simulink model "mppt_zero_handled"  (R2022a)
settings: Solver=VariableStepAuto  StartTime=0.0  StopTime=1.5  RelTol=1e-3
undefined symbols (not defined in the file or in its folder): DiscIntNeverNeededParam
libraries: simulink x5, spsSeriesRLCBranchLib x4, spsDiodeLib x2, fuzblock x2, spsIGBTDiodeLib x1, spsCurrentMeasurementLib x1, spsPVArrayLib x1, spsPWMGeneratorDCDCLib x1, spsVoltageMeasurementLib x1, spspowerguiLib x1
settings Model: Creator=IshaanKarnik  LastModifiedBy=IshaanKarnik
settings DebuggingCC: UnconnectedInputMsg=warning  UnconnectedOutputMsg=warning  UnconnectedLineMsg=warning
settings RTWCC: DLArmComputeVersion=19.05

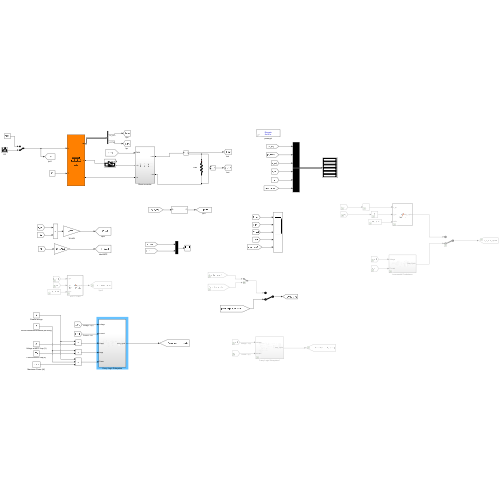
[thumbnail: Simulink's stored preview of the top-level diagram]
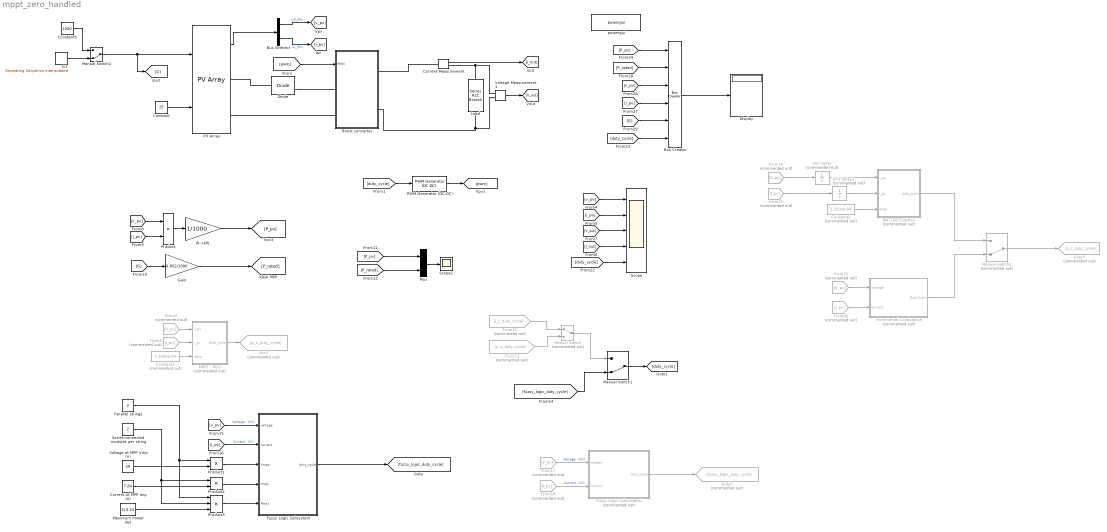
== system mppt_zero_handled ==
  Boost converter : Subsystem
  Bus Creator : BusCreator  Inputs=6
  Bus Selector : BusSelector  OutputSignals=V_PV,I_PV
  Constant : Constant  Value=25
  Constant1 : Constant  Commented=on  Value=1.2500e-04
  Constant2 : Constant  Commented=on  Value=1.2500e-04
  Constant3 : Constant  Value=1000
  Current Measurement : spsCurrentMeasurementLib/Current Measurement  PhasorSimulation=off  OutputType=Complex  PSBequivalent=0
  Current at MPP Imp (A) : Constant  Value=7.84
  Diode : spsDiodeLib/Diode  Ron=0.001  Lon=0  Vf=0.8  IC=0  UseSnubber=0  Rs=500  Cs=250e-9  Measurements=on
  Display : Display
  From13 : From  Commented=on  GotoTag=p_o_duty_cycle
  From{2,17,19,25} (4 alike) : From  Commented=on  GotoTag=V_pv
  From{3,18,20,30} (4 alike) : From  Commented=on  GotoTag=I_pv
  From21 : From  Commented=on  GotoTag=i_c_duty_cycle
  Fuzzy Logic Subsystem : Subsystem
  Fuzzy Logic Subsystem1 : Subsystem  Commented=on
  G2 : simulink/Sources/Repeating Sequence Interpolated  OutValues=[0 0 300 300 500 500 1000 1000 500 500 0 0].'  TimeValues=[0 0.25 0.2501 0.5 0.501 0.75 0.7501 1 1.01 1.25 1.2501 1.5].'  LookUpMeth=Interpolation-Use End Values  tsamp=0.01  OutMin=[]  OutMax=[]  OutDataTypeStr=double  OutputDataTypeScalingMode=double  OutDataType=fixdt(0,8)  OutScaling=2^-10
  Gain : Gain  Gain=0.852/1000
  Goto2 : Goto  Commented=on  GotoTag=fuzzy_logic_duty_cycle
  Goto4 : Goto  Commented=on  GotoTag=i_c_duty_cycle
  Incremental Condutance : Subsystem  Commented=on
  Load : spsSeriesRLCBranchLib/Series RLC Branch  LConnTagsString=__new0  RConnTagsString=__new0  BranchType=R  Resistance=20  Inductance=1e-3  SetiL0=off  InitialCurrent=0  Capacitance=100e-6  Setx0=off  InitialVoltage=0  Measurements=None
  MATLAB Function : MATLAB Function  Commented=on  TreatAsAtomicUnit=on
  MPPT - P&O : MATLAB Function  Commented=on  TreatAsAtomicUnit=on
  Manual Switch : ManualSwitch  Commented=on
  Manual Switch1 : ManualSwitch  CurrentSetting=0
  Manual Switch2 : ManualSwitch  CurrentSetting=0
  Manual Switch3 : ManualSwitch  Commented=on  CurrentSetting=0
  Maximum Power (W) : Constant  Value=213.15
  Mux : Mux  Inputs=2
  PV Array : spsPVArrayLib/PV Array  Npar=2  Nser=2  PlotType=array @ 25 deg.C & specified irradiances  S_vec="[ 1000  500  100 ]"  Temp_C_vec="[ 45 25  ]"  ModuleName=User-defined  PlotWhenSelected=off  Pm=213.15  Ncell=60  Voc=36.3  Isc=7.84  Vm=29  Im=7.35  beta_Voc_pc=-0.36099  alpha_Isc_pc=0.102  beta_Voc=-0.13104  alpha_Isc=0.0079968  IL=7.8654  I0=2.9273e-10  nI=0.98119  Rsh=313.0553  Rs=0.39381  RobustModel=off  RobustCellTemperature=313.3991  BAL=off  Tc=1e-6  Tfilter=5e-5
  PWM Generator (DC-DC) : spsPWMGeneratorDCDCLib/PWM Generator (DC-DC)  Fsw=5000  Ts=5e-6
  Parallel strings : Constant  Value=2
  Product : Product
  Product1 : Product
  Product2 : Product
  Product3 : Product  Inputs=3
  Scope : Scope  NumInputPorts=5
  Scope1 : Scope
  Series-connected modules per string : Constant  Value=2
  Unit Delay : UnitDelay  Commented=on  SampleTime=100e-6  HasFrameUpgradeWarning=on
  Unit Delay1 : UnitDelay  Commented=on  SampleTime=100e-6  HasFrameUpgradeWarning=on
  Voltage Measurement1 : spsVoltageMeasurementLib/Voltage Measurement  PhasorSimulation=off  OutputType=Complex  PSBequivalent=0
  Voltage at MPP Vmp (V) : Constant  Value=29
  Vpv2 : Goto  Commented=on  GotoTag=p_o_duty_cycle
  W->kW : Gain  Gain=1/1000
  powergui : spspowerguiLib/powergui  Priority=1  SimulationMode=Discrete  SampleTime=5e-6  frequency=60  Iterations=50  frequencyindice=0  Pbase=100e6  ErrMax=1e-4  UnitsV=kV  UnitsW=MW  buscounter=0  FunctionMessages=off  echomessages=off  EnableUseOfTLC=off  CurrentSourceSwitches=off  DisableSnubberDevices=off  DisableRonSwitches=off  DisableVfSwitches=off  DisplayEquations=off  AutomaticDiscreteSolvers=off  SolverType=Tustin/Backward Euler (TBE)  Interpol=off  ExternalGateDelay=off  methode=off  Ts=100  x0status=blocks  SPID=on  SwTol=0  HookPort=off  NonlinearTolerance=1e-4  nMaxIteration=100  ContinueOnMaxIteration=off  RestoreLinks=warning  ResistiveCurrentMeasurement=off  Frange=[0:2:500]  Ylog=off  Xlog=on  ShowGrid=off  save=off  variable=ZData  structure=0  ZoomFFT=off  StartTime=0.0  cycles=1  DisplayStyle=1  fundamental=60  FreqAxis=off  MaxFrequency=1000  frequencyindicesteady=1  RmsSteady=1  display=off
  wires:
  [I_out] -> Scope/4
  Unit Delay/1 -> MATLAB Function/1(v_pv)
  From25/1 -> Incremental Condutance/1(Voltage)
  [v_pv] -> Scope/1
  Manual Switch1/1 -> [duty_cycle]
  [duty_cycle] -> Scope/5
  [fuzzy_logic_duty_cycle] -> Manual Switch1/2
  Constant3/1 -> Manual Switch2/1
  From19/1 -> Unit Delay/1
  Bus Creator/1 -> Display/1
  Bus Selector/1 -> [v_pv]  "<V_PV>"
  Manual Switch2/1 -> [G], PV Array/1
  [v_pv] -> Product/1
  [G] -> Bus Creator/5
  Gain/1 -> [P_rated]
  [P_pv] -> Mux/1
  MPPT - P&O/1(duty_cycle) -> Vpv2/1
  [G] -> Gain/1
  [i_pv] -> Scope/2
  [P_rated] -> Bus Creator/2
  [duty_cycle] -> PWM Generator (DC-DC)/1
  W->kW/1 -> [P_pv]
  Constant/1 -> PV Array/2
  Bus Selector/2 -> [i_pv]  "<I_PV>"
  [i_pv] -> Product/2
  Product/1 -> W->kW/1
  Constant1/1 -> MPPT - P&O/3(delta)
  From13/1 -> Manual Switch/2
  Mux/1 -> Scope1/1
  [v_pv] -> Fuzzy Logic Subsystem/1(voltage)  "Voltage - V(n)"
  From3/1 -> MPPT - P&O/2(i_pv)
  From17/1 -> Fuzzy Logic Subsystem1/1(voltage)  "Voltage - V(n)"
  G2/1 -> Manual Switch2/2
  From21/1 -> Manual Switch/1
  Constant2/1 -> MATLAB Function/3(delta)
  From30/1 -> Incremental Condutance/2(Current)
  From2/1 -> MPPT - P&O/1(v_pv)
  Fuzzy Logic Subsystem1/1(duty_cycle) -> Goto2/1
  [pwm] -> Boost converter/1(PWM)
  Voltage Measurement1/1 -> [V_out]
  Unit Delay1/1 -> MATLAB Function/2(i_pv)
  MATLAB Function/1(duty_cycle) -> Manual Switch3/1
  [V_out] -> Scope/3
  [i_pv] -> Bus Creator/4
  [v_pv] -> Bus Creator/3
  Current Measurement/1 -> [I_out]
  From18/1 -> Fuzzy Logic Subsystem1/2(current)  "Current - I(n)"
  [P_rated] -> Mux/2
  PV Array/1 -> Bus Selector/1
  From20/1 -> Unit Delay1/1
  Manual Switch3/1 -> Goto4/1
  PWM Generator (DC-DC)/1 -> [pwm]
  [duty_cycle] -> Bus Creator/6
  [i_pv] -> Fuzzy Logic Subsystem/2(current)  "Current - I(n)"
  Incremental Condutance/1(Duty Cycle) -> Manual Switch3/2
  Manual Switch/1 -> Manual Switch1/1
  [P_pv] -> Bus Creator/1
  Fuzzy Logic Subsystem/1(duty_cycle) -> [fuzzy_logic_duty_cycle]
  Product1/1 -> Fuzzy Logic Subsystem/3(Vmpp)
  Voltage at MPP Vmp (V)/1 -> Product1/2
  Product2/1 -> Fuzzy Logic Subsystem/4(Impp)
  Current at MPP Imp (A)/1 -> Product2/2
  Product3/1 -> Fuzzy Logic Subsystem/5(Pmax)
  Series-connected modules per string/1 -> Product3/2, Product2/1
  Parallel strings/1 -> Product3/1, Product1/1
  Maximum Power (W)/1 -> Product3/3
  connections:
  Boost converter/RConn2 -- Voltage Measurement1/LConn2 -- Load/RConn1
  Current Measurement/RConn1 -- Voltage Measurement1/LConn1 -- Load/LConn1
  PV Array/RConn2 -- Boost converter/LConn2
  Current Measurement/LConn1 -- Boost converter/RConn1
  Diode/RConn1 -- Boost converter/LConn1
  Diode/LConn1 -- PV Array/RConn1

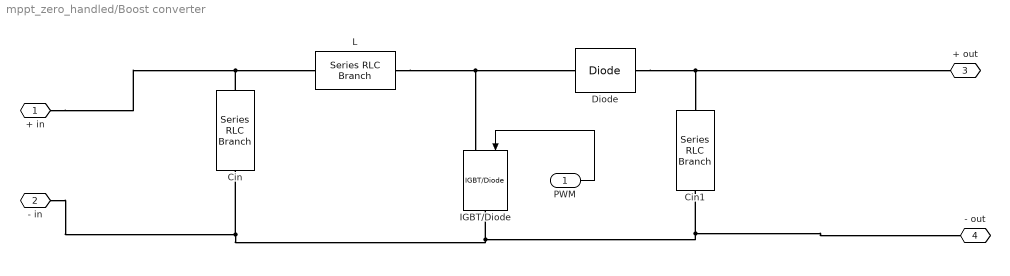
== system mppt_zero_handled/Boost converter ==
  PWM : Inport
  Cin : spsSeriesRLCBranchLib/Series RLC Branch  LConnTagsString=__new0  RConnTagsString=__new0  BranchType=RC  Resistance=1e-3  Inductance=1e-3  SetiL0=off  InitialCurrent=0  Capacitance=50e-6  Setx0=off  InitialVoltage=0  Measurements=None
  Cin1 : spsSeriesRLCBranchLib/Series RLC Branch  LConnTagsString=__new0  RConnTagsString=__new0  BranchType=RC  Resistance=1e-4  Inductance=1e-3  SetiL0=off  InitialCurrent=0  Capacitance=10e-6  Setx0=off  InitialVoltage=0  Measurements=None
  Diode : spsDiodeLib/Diode  Ron=0.001  Lon=0  Vf=0.8  IC=0  UseSnubber=0  Rs=500  Cs=250e-9  Measurements=off
  IGBT/Diode : spsIGBTDiodeLib/IGBT//Diode  Ron=1e-3  Rs=1e5  Cs=inf  Measurements=off
  L : spsSeriesRLCBranchLib/Series RLC Branch  LConnTagsString=__new0  RConnTagsString=__new0  BranchType=RL  Resistance=0.1  Inductance=2e-3  SetiL0=off  InitialCurrent=0  Capacitance=100e-6  Setx0=off  InitialVoltage=0  Measurements=None
  + in : PMIOPort  Side=Left
  - in : PMIOPort  Port=2  Side=Left
  + out : PMIOPort  Port=3  Side=Right
  - out : PMIOPort  Port=4  Side=Right
  wires:
  PWM/1 -> IGBT/Diode/1
  connections:
  Cin/LConn1 -- + in/RConn1 -- L/RConn1
  - in/RConn1 -- Cin/RConn1 -- - out/RConn1 -- Cin1/RConn1 -- IGBT/Diode/RConn1
  L/LConn1 -- Diode/LConn1 -- IGBT/Diode/LConn1
  Diode/RConn1 -- + out/RConn1 -- Cin1/LConn1

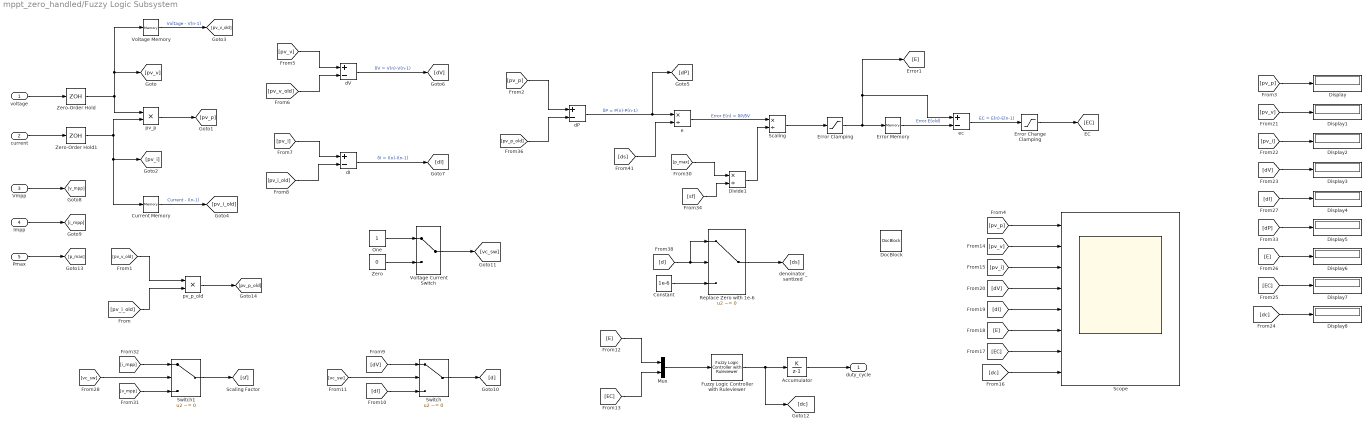
== system mppt_zero_handled/Fuzzy Logic Subsystem ==
  voltage : Inport
  current : Inport  Port=2
  Vmpp : Inport  Port=3
  Impp : Inport  Port=4
  Pmax : Inport  Port=5
  Accumulator : DiscreteIntegrator  IntegratorMethod=Accumulation: Forward Euler  gainval=0.1  InitialCondition=0.3  SampleTime=-1  LimitOutput=on  UpperSaturationLimit=1  LowerSaturationLimit=0  ICPrevOutput=DiscIntNeverNeededParam  ICPrevScaledInput=DiscIntNeverNeededParam
  Constant : Constant  Value=1e-6
  Current Memory : Memory
  Display{,1..8} (9 alike) : Display
  Divide1 : Product  Inputs=*/
  DocBlock : simulink/Model-Wide Utilities/DocBlock  DocumentType=Text
      content=|
      | Error E(n) = δP/δV or
      | Error E(n) = δP/δI
      | Depending on the manual switch setting
  Error Change Clamping : Saturate  UpperLimit=2  LowerLimit=-2
  Error Clamping : Saturate  UpperLimit=1  LowerLimit=-1
  Error Memory : Memory
  Fuzzy Logic Controller with Ruleviewer : fuzblock/Fuzzy Logic  Controller  with Ruleviewer  fismatrix=fuzzy_mppt  Ts=0.1
  Mux : Mux  Inputs=2
  One : Constant  OutDataTypeStr=Inherit: Inherit via back propagation
  Replace Zero with 1e-6 : Switch  Criteria=u2 ~= 0  SaturateOnIntegerOverflow=off  InputSameDT=off
  Scaling : Product  Inputs=*/
  Scope : Scope  NumInputPorts=8
  Switch : Switch  Criteria=u2 ~= 0  SaturateOnIntegerOverflow=off  InputSameDT=off
  Switch1 : Switch  Criteria=u2 ~= 0  SaturateOnIntegerOverflow=off  InputSameDT=off
  Voltage Current Switch : ManualSwitch
  Voltage Memory : Memory
  Zero : Constant  Value=0  OutDataTypeStr=Inherit: Inherit via back propagation
  Zero-Order Hold : ZeroOrderHold  SampleTime=-1
  Zero-Order Hold1 : ZeroOrderHold  SampleTime=-1
  dI : Sum  Inputs=+-
  dP : Sum  Inputs=+-
  dV : Sum  Inputs=+-
  e : Product  Inputs=*/
  ec : Sum  Inputs=+-
  pv_p : Product
  pv_p_old : Product
  duty_cycle : Outport
  wires:
  ec/1 -> Error Change Clamping/1  "EC = E(n)-E(n-1)"
  dP/1 -> [dP], e/1  "δP = P(n)-P(n-1)"
  [dI] -> Display4/1
  dV/1 -> [dV]  "δV = V(n)-V(n-1)"
  [EC] -> Display7/1
  Voltage Memory/1 -> [pv_v_old]  "Voltage - V(n-1)"
  [pv_v_old] -> dV/2
  [pv_i_old] -> dI/2
  [pv_v] -> dV/1
  [EC] -> Mux/2
  [pv_i] -> Display2/1
  dI/1 -> [dI]  "δI = I(n)-I(n-1)"
  Error Memory/1 -> ec/2  "Error E(old)"
  [pv_p] -> Scope/1
  [pv_p] -> Display/1
  [dV] -> Scope/4
  [pv_i] -> Scope/3
  [E] -> Display6/1
  [pv_v] -> Scope/2
  [dI] -> Scope/5
  [dc] -> Display8/1
  [E] -> Mux/1
  Current Memory/1 -> [pv_i_old]  "Current - I(n-1)"
  [dc] -> Scope/8
  [EC] -> Scope/7
  [E] -> Scope/6
  [pv_i] -> dI/1
  [dV] -> Display3/1
  [pv_v] -> Display1/1
  current/1 -> Zero-Order Hold1/1
  voltage/1 -> Zero-Order Hold/1
  Zero-Order Hold1/1 -> Current Memory/1, [pv_i], pv_p/2
  Zero-Order Hold/1 -> pv_p/1, Voltage Memory/1, [pv_v]
  [dP] -> Display5/1
  pv_p/1 -> [pv_p]
  [pv_v_old] -> pv_p_old/1
  [pv_i_old] -> pv_p_old/2
  pv_p_old/1 -> [pv_p_old]
  [pv_p_old] -> dP/2
  [pv_p] -> dP/1
  Error Change Clamping/1 -> [EC]
  Vmpp/1 -> [v_mpp]
  Impp/1 -> [i_mpp]
  Pmax/1 -> [p_max]
  e/1 -> Scaling/1  "Error E(n) = δP/δV"
  [sf] -> Divide1/2
  Mux/1 -> Fuzzy Logic Controller with Ruleviewer/1
  [p_max] -> Divide1/1
  Constant/1 -> Replace Zero with 1e-6/3
  [d] -> Replace Zero with 1e-6/2, Replace Zero with 1e-6/1
  Replace Zero with 1e-6/1 -> [ds]
  [ds] -> e/2
  Scaling/1 -> Error Clamping/1
  Error Clamping/1 -> ec/1, [E], Error Memory/1
  Accumulator/1 -> duty_cycle/1
  Fuzzy Logic Controller with Ruleviewer/1 -> [dc], Accumulator/1
  Switch/1 -> [d]
  [dV] -> Switch/1
  [dI] -> Switch/3
  Switch1/1 -> [sf]
  Zero/1 -> Voltage Current Switch/2
  One/1 -> Voltage Current Switch/1
  Voltage Current Switch/1 -> [vc_sw]
  [vc_sw] -> Switch1/2
  [vc_sw] -> Switch/2
  Divide1/1 -> Scaling/2
  [v_mpp] -> Switch1/3
  [i_mpp] -> Switch1/1

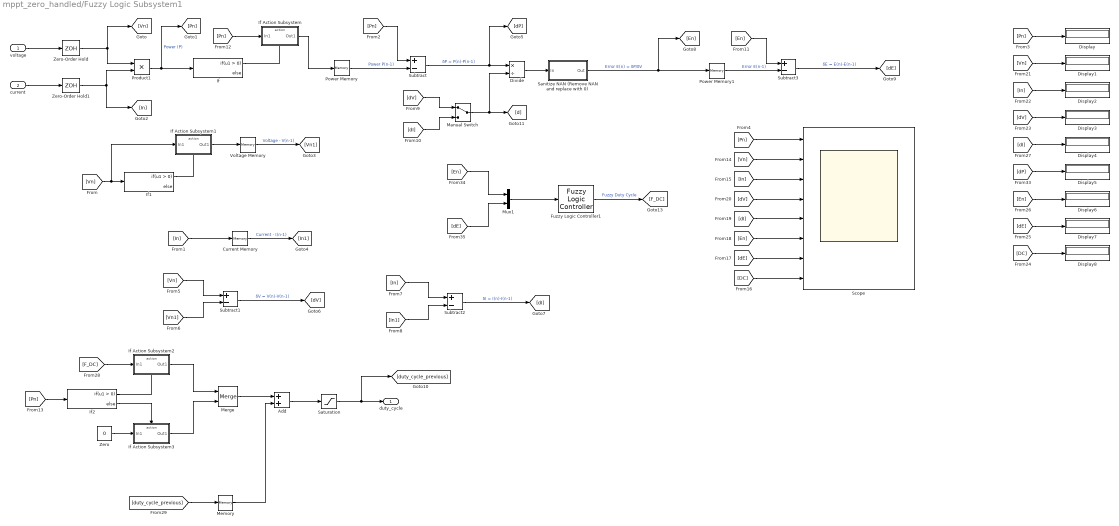
== system mppt_zero_handled/Fuzzy Logic Subsystem1 ==
  voltage : Inport
  current : Inport  Port=2
  Add : Sum
  Current Memory : Memory
  Display{,1..8} (9 alike) : Display
  Divide : Product  Inputs=*/
  Fuzzy Logic Controller1 : fuzblock/Fuzzy Logic  Controller  FIS=fuzzy_mppt  OutputSampleNumber=101  DataType=double  FuzzifiedInputs=off  RuleFiringStrengths=off  RuleOutputs=off  AggregatedOutputs=off  SimulateUsing=Interpreted execution  OutOfRangeInputValueMessage=warning  NoRuleFiredMessage=warning  EmptyOutputFuzzySetMessage=warning
  If : If
  If Action Subsystem : Subsystem  TreatAsAtomicUnit=on
  If Action Subsystem1 : Subsystem  TreatAsAtomicUnit=on
  If Action Subsystem2 : Subsystem  TreatAsAtomicUnit=on
  If Action Subsystem3 : Subsystem  TreatAsAtomicUnit=on
  If1 : If
  If2 : If
  Manual Switch : ManualSwitch
  Memory : Memory
  Merge : Merge
  Mux1 : Mux  Inputs=2
  Power Memory : Memory
  Power Memory1 : Memory
  Product1 : Product
  Sanitize NAN (Remove NAN and replace with 0) : Subsystem
  Saturation : Saturate  UpperLimit=0.85  LowerLimit=0
  Scope : Scope  NumInputPorts=8
  Subtract{,1..3} (4 alike) : Sum  Inputs=+-
  Voltage Memory : Memory
  Zero : Constant  Value=0  OutDataTypeStr=Inherit: Inherit via back propagation
  Zero-Order Hold : ZeroOrderHold  SampleTime=-1
  Zero-Order Hold1 : ZeroOrderHold  SampleTime=-1
  duty_cycle : Outport
  wires:
  Sanitize NAN (Remove NAN and replace with 0)/1(Out) -> [En], Power Memory1/1  "Error E(n) = δP/δV"
  Subtract3/1 -> [dE]  "δE = E(n)-E(n-1)"
  Subtract/1 -> [dP], Divide/1  "δP = P(n)-P(n-1)"
  [Pn] -> Subtract/1
  [dI] -> Display4/1
  Subtract1/1 -> [dV]  "δV = V(n)-V(n-1)"
  [dE] -> Display7/1
  Manual Switch/1 -> [d], Divide/2
  Voltage Memory/1 -> [Vn1]  "Voltage - V(n-1)"
  [Vn1] -> Subtract1/2
  [In1] -> Subtract2/2
  [Vn] -> Subtract1/1
  Power Memory/1 -> Subtract/2  "Power P(n-1)"
  [In] -> Display2/1
  Subtract2/1 -> [dI]  "δI = I(n)-I(n-1)"
  Power Memory1/1 -> Subtract3/2  "Error E(n-1)"
  [dV] -> Manual Switch/1
  [Pn] -> Scope/1
  [Pn] -> Display/1
  [dV] -> Scope/4
  [In] -> Scope/3
  [En] -> Display6/1
  [Vn] -> Scope/2
  [dI] -> Scope/5
  [En] -> Subtract3/1
  [DC] -> Display8/1
  Current Memory/1 -> [In1]  "Current - I(n-1)"
  [DC] -> Scope/8
  [dE] -> Scope/7
  [En] -> Scope/6
  [In] -> Subtract2/1
  [dV] -> Display3/1
  [dI] -> Manual Switch/2
  [Vn] -> Display1/1
  Memory/1 -> Add/2
  [duty_cycle_previous] -> Memory/1
  current/1 -> Zero-Order Hold1/1
  voltage/1 -> Zero-Order Hold/1
  Zero-Order Hold1/1 -> [In], Product1/2
  Zero-Order Hold/1 -> Product1/1, [Vn]
  [dP] -> Display5/1
  [En] -> Mux1/1
  Fuzzy Logic Controller1/1 -> [F_DC]  "Fuzzy Duty Cycle"
  Mux1/1 -> Fuzzy Logic Controller1/1
  [dE] -> Mux1/2
  Add/1 -> Saturation/1
  Saturation/1 -> [duty_cycle_previous], duty_cycle/1
  [In] -> Current Memory/1
  Divide/1 -> Sanitize NAN (Remove NAN and replace with 0)/1(In)
  Product1/1 -> If/1, [Pn]  "Power (P)"
  If/1 -> If Action Subsystem/Action
  If Action Subsystem/1(Out1) -> Power Memory/1
  [Pn] -> If Action Subsystem/1(In1)
  [Vn] -> If Action Subsystem1/1(In1), If1/1
  If Action Subsystem1/1(Out1) -> Voltage Memory/1
  If1/1 -> If Action Subsystem1/Action
  If2/1 -> If Action Subsystem2/Action
  [Pn] -> If2/1
  [F_DC] -> If Action Subsystem2/1(In1)
  Merge/1 -> Add/1
  If Action Subsystem2/1(Out1) -> Merge/1
  If2/2 -> If Action Subsystem3/Action
  If Action Subsystem3/1(Out1) -> Merge/2
  Zero/1 -> If Action Subsystem3/1(In1)

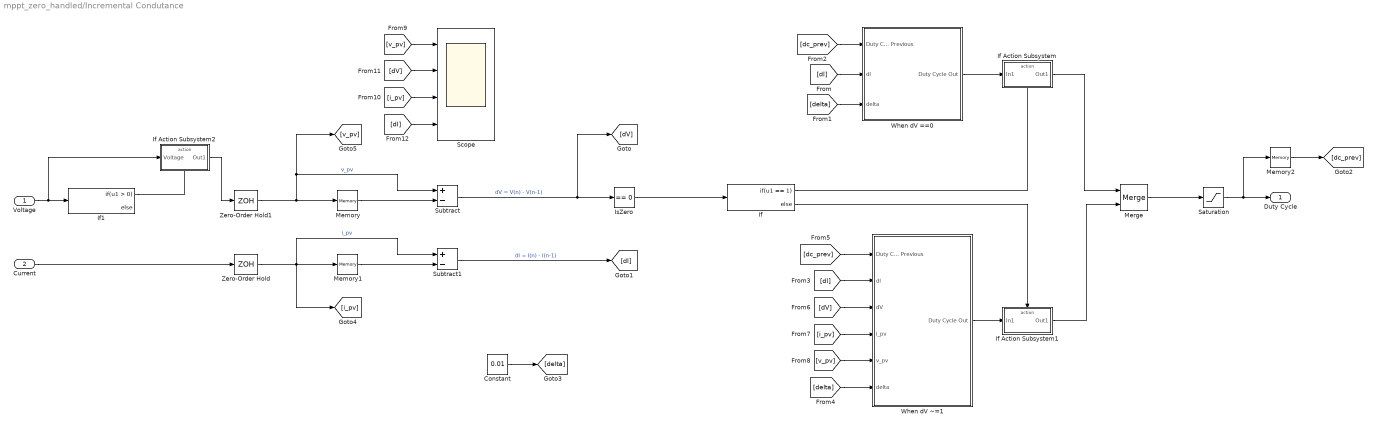
== system mppt_zero_handled/Incremental Condutance ==
  Voltage : Inport
  Current : Inport  Port=2
  Constant : Constant  Value=0.01
  If : If  IfExpression=u1 == 1
  If Action Subsystem : Subsystem  TreatAsAtomicUnit=on
  If Action Subsystem1 : Subsystem  TreatAsAtomicUnit=on
  If Action Subsystem2 : Subsystem  TreatAsAtomicUnit=on
  If1 : If
  IsZero : simulink/Logic and Bit Operations/Compare To Zero  relop===  OutDataTypeStr=boolean
  Memory : Memory
  Memory1 : Memory
  Memory2 : Memory
  Merge : Merge
  Saturation : Saturate  UpperLimit=0.85  LowerLimit=0
  Scope : Scope  NumInputPorts=4
  Subtract : Sum  Inputs=+-
  Subtract1 : Sum  Inputs=+-
  When dV ==0 : Subsystem
  When dV ~=1 : Subsystem
  Zero-Order Hold : ZeroOrderHold  SampleTime=-1
  Zero-Order Hold1 : ZeroOrderHold  SampleTime=-1
  Duty Cycle : Outport
  wires:
  Zero-Order Hold1/1 -> [v_pv], Subtract/1, Memory/1  "v_pv"
  Zero-Order Hold/1 -> [i_pv], Subtract1/1, Memory1/1  "i_pv"
  Memory/1 -> Subtract/2
  Memory1/1 -> Subtract1/2
  Subtract/1 -> [dV], IsZero/1  "dV = V(n) - V(n-1)"
  Subtract1/1 -> [dI]  "dI = I(n) - I(n-1)"
  IsZero/1 -> If/1
  If/2 -> If Action Subsystem1/Action
  If/1 -> If Action Subsystem/Action
  If Action Subsystem1/1(Out1) -> Merge/2
  Saturation/1 -> Memory2/1, Duty Cycle/1
  Memory2/1 -> [dc_prev]
  Constant/1 -> [delta]
  If Action Subsystem/1(Out1) -> Merge/1
  When dV ==0/1(Duty Cycle Out) -> If Action Subsystem/1(In1)
  [dI] -> When dV ==0/2(dI)
  [delta] -> When dV ==0/3(delta)
  [dc_prev] -> When dV ==0/1(Duty Cycle Previous)
  When dV ~=1/1(Duty Cycle Out) -> If Action Subsystem1/1(In1)
  Merge/1 -> Saturation/1
  [dc_prev] -> When dV ~=1/1(Duty Cycle Previous)
  [dI] -> When dV ~=1/2(dI)
  [dV] -> When dV ~=1/3(dV)
  [delta] -> When dV ~=1/6(delta)
  [i_pv] -> When dV ~=1/4(i_pv)
  [v_pv] -> When dV ~=1/5(v_pv)
  [v_pv] -> Scope/1
  [dV] -> Scope/2
  [i_pv] -> Scope/3
  [dI] -> Scope/4
  Voltage/1 -> If Action Subsystem2/1(Voltage), If1/1
  If1/1 -> If Action Subsystem2/Action
  If Action Subsystem2/1(Out1) -> Zero-Order Hold1/1
  Current/1 -> Zero-Order Hold/1

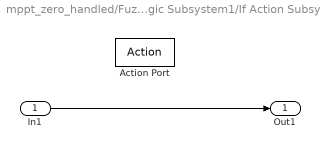
== system mppt_zero_handled/Fuzzy Logic Subsystem1/If Action Subsystem ==
  In1 : Inport
  Action Port : ActionPort
  Out1 : Outport
  wires:
  In1/1 -> Out1/1

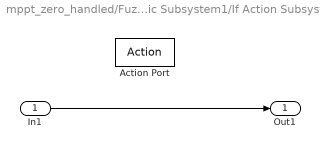
== system mppt_zero_handled/Fuzzy Logic Subsystem1/If Action Subsystem1 ==
  In1 : Inport
  Action Port : ActionPort
  Out1 : Outport
  wires:
  In1/1 -> Out1/1

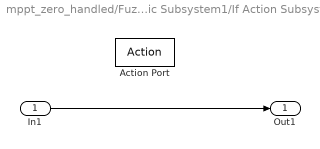
== system mppt_zero_handled/Fuzzy Logic Subsystem1/If Action Subsystem2 ==
  In1 : Inport
  Action Port : ActionPort
  Out1 : Outport
  wires:
  In1/1 -> Out1/1

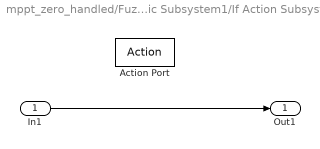
== system mppt_zero_handled/Fuzzy Logic Subsystem1/If Action Subsystem3 ==
  In1 : Inport
  Action Port : ActionPort
  Out1 : Outport
  wires:
  In1/1 -> Out1/1

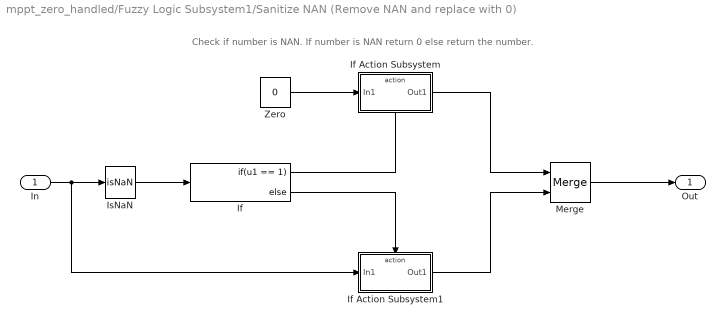
== system mppt_zero_handled/Fuzzy Logic Subsystem1/Sanitize NAN (Remove NAN and replace with 0) ==
  note: Check if number is NAN. If number is NAN return 0 else return the number.
  In : Inport
  If : If  IfExpression=u1 == 1
  If Action Subsystem : Subsystem  TreatAsAtomicUnit=on
  If Action Subsystem1 : Subsystem  TreatAsAtomicUnit=on
  IsNaN : RelationalOperator  Operator=isNaN  OutDataTypeStr=boolean  RndMeth=Simplest  InputSameDT=off
  Merge : Merge  InitialOutput=[0]
  Zero : Constant  Value=0  OutDataTypeStr=Inherit: Inherit via back propagation
  Out : Outport
  wires:
  If/1 -> If Action Subsystem/Action
  If Action Subsystem/1(Out1) -> Merge/1
  Zero/1 -> If Action Subsystem/1(In1)
  IsNaN/1 -> If/1
  In/1 -> If Action Subsystem1/1(In1), IsNaN/1
  Merge/1 -> Out/1
  If Action Subsystem1/1(Out1) -> Merge/2
  If/2 -> If Action Subsystem1/Action

== system mppt_zero_handled/Incremental Condutance/If Action Subsystem ==
  In1 : Inport
  Action Port : ActionPort
  Out1 : Outport
  wires:
  In1/1 -> Out1/1

== system mppt_zero_handled/Incremental Condutance/If Action Subsystem1 ==
  In1 : Inport
  Action Port : ActionPort
  Out1 : Outport
  wires:
  In1/1 -> Out1/1

== system mppt_zero_handled/Incremental Condutance/If Action Subsystem2 ==
  Voltage : Inport
  Action Port : ActionPort
  Out1 : Outport
  wires:
  Voltage/1 -> Out1/1

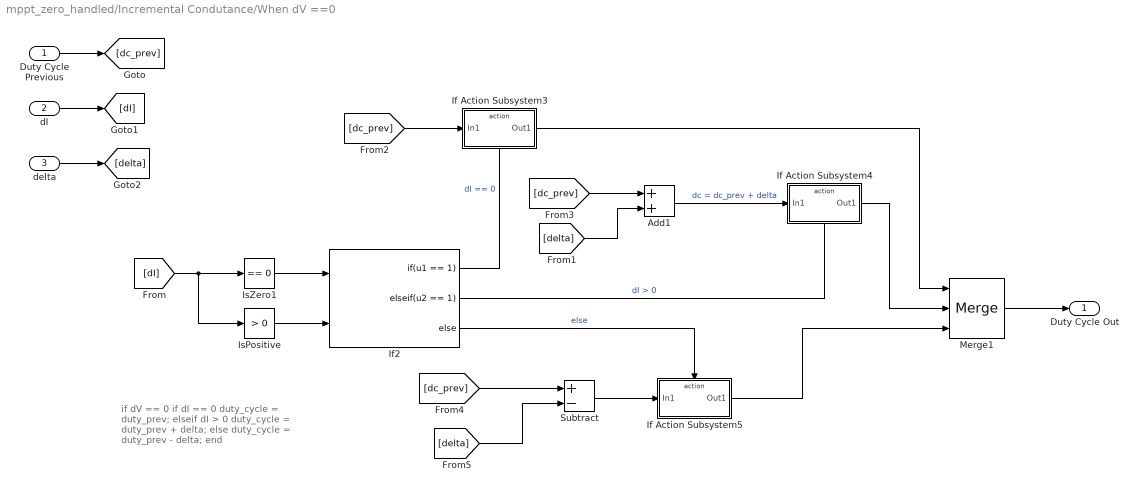
== system mppt_zero_handled/Incremental Condutance/When dV ==0 ==
  note: if dV == 0
      |     if dI == 0
      |         duty_cycle = duty_prev;
      |     elseif dI > 0
      |         duty_cycle = duty_prev + delta;
      |     else
      |         duty_cycle = duty_prev - delta;
      | end
  Duty Cycle Previous : Inport
  dI : Inport  Port=2
  delta : Inport  Port=3
  Add1 : Sum
  If Action Subsystem3 : Subsystem  TreatAsAtomicUnit=on
  If Action Subsystem4 : Subsystem  TreatAsAtomicUnit=on
  If Action Subsystem5 : Subsystem  TreatAsAtomicUnit=on
  If2 : If  NumInputs=2  IfExpression=u1 == 1  ElseIfExpressions=u2 == 1
  IsPositive : simulink/Logic and Bit Operations/Compare To Zero  relop=>  OutDataTypeStr=boolean
  IsZero1 : simulink/Logic and Bit Operations/Compare To Zero  relop===  OutDataTypeStr=boolean
  Merge1 : Merge  Inputs=3
  Subtract : Sum  Inputs=+-
  Duty Cycle Out : Outport
  wires:
  [dI] -> IsPositive/1, IsZero1/1
  IsZero1/1 -> If2/1
  Add1/1 -> If Action Subsystem4/1(In1)  "dc = dc_prev + delta"
  Subtract/1 -> If Action Subsystem5/1(In1)
  If2/3 -> If Action Subsystem5/Action  "else"
  [dc_prev] -> Add1/1
  If2/2 -> If Action Subsystem4/Action  "dI > 0"
  [dc_prev] -> Subtract/1
  If Action Subsystem3/1(Out1) -> Merge1/1
  [delta] -> Subtract/2
  IsPositive/1 -> If2/2
  Merge1/1 -> Duty Cycle Out/1
  If Action Subsystem5/1(Out1) -> Merge1/3
  If Action Subsystem4/1(Out1) -> Merge1/2
  [dc_prev] -> If Action Subsystem3/1(In1)
  If2/1 -> If Action Subsystem3/Action  "dI == 0"
  Duty Cycle Previous/1 -> [dc_prev]
  dI/1 -> [dI]
  delta/1 -> [delta]
  [delta] -> Add1/2

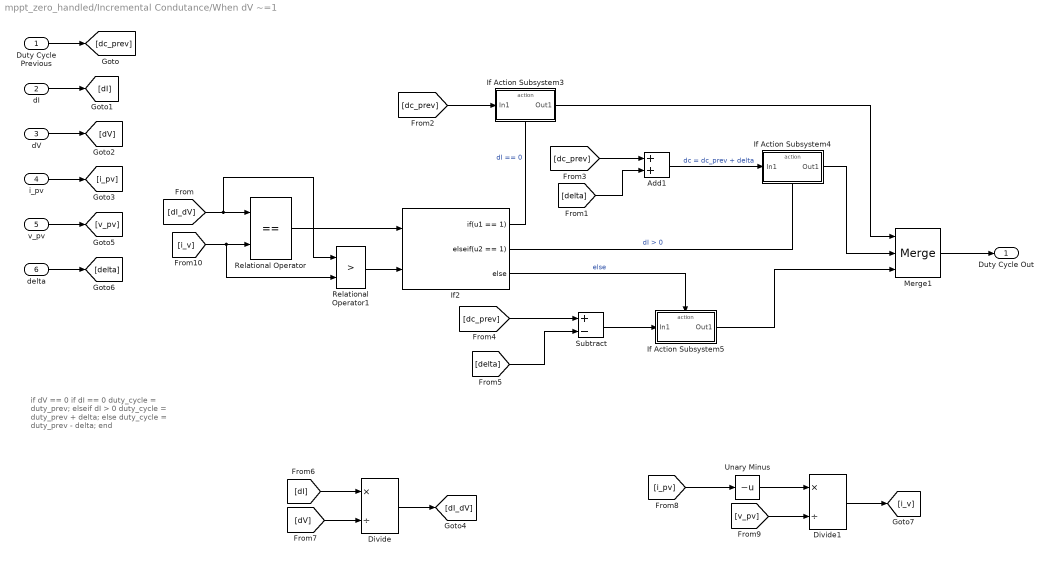
== system mppt_zero_handled/Incremental Condutance/When dV ~=1 ==
  note: if dV == 0
      |     if dI == 0
      |         duty_cycle = duty_prev;
      |     elseif dI > 0
      |         duty_cycle = duty_prev + delta;
      |     else
      |         duty_cycle = duty_prev - delta;
      | end
  Duty Cycle Previous : Inport
  dI : Inport  Port=2
  dV : Inport  Port=3
  i_pv : Inport  Port=4
  v_pv : Inport  Port=5
  delta : Inport  Port=6
  Add1 : Sum
  Divide : Product  Inputs=*/
  Divide1 : Product  Inputs=*/
  If Action Subsystem3 : Subsystem  TreatAsAtomicUnit=on
  If Action Subsystem4 : Subsystem  TreatAsAtomicUnit=on
  If Action Subsystem5 : Subsystem  TreatAsAtomicUnit=on
  If2 : If  NumInputs=2  IfExpression=u1 == 1  ElseIfExpressions=u2 == 1
  Merge1 : Merge  Inputs=3
  Relational Operator : RelationalOperator  Operator===  OutDataTypeStr=boolean  RndMeth=Simplest  InputSameDT=off
  Relational Operator1 : RelationalOperator  Operator=>  OutDataTypeStr=boolean  RndMeth=Simplest  InputSameDT=off
  Subtract : Sum  Inputs=+-
  Unary Minus : UnaryMinus
  Duty Cycle Out : Outport
  wires:
  [delta] -> Add1/2
  dV/1 -> [dV]
  dI/1 -> [dI]
  Duty Cycle Previous/1 -> [dc_prev]
  If2/1 -> If Action Subsystem3/Action  "dI == 0"
  [dc_prev] -> If Action Subsystem3/1(In1)
  If Action Subsystem4/1(Out1) -> Merge1/2
  If Action Subsystem5/1(Out1) -> Merge1/3
  Merge1/1 -> Duty Cycle Out/1
  [delta] -> Subtract/2
  If Action Subsystem3/1(Out1) -> Merge1/1
  [dc_prev] -> Subtract/1
  If2/2 -> If Action Subsystem4/Action  "dI > 0"
  [dc_prev] -> Add1/1
  If2/3 -> If Action Subsystem5/Action  "else"
  Subtract/1 -> If Action Subsystem5/1(In1)
  Add1/1 -> If Action Subsystem4/1(In1)  "dc = dc_prev + delta"
  i_pv/1 -> [i_pv]
  [dI] -> Divide/1
  [dV] -> Divide/2
  Divide/1 -> [dI_dV]
  v_pv/1 -> [v_pv]
  delta/1 -> [delta]
  [v_pv] -> Divide1/2
  [i_pv] -> Unary Minus/1
  Unary Minus/1 -> Divide1/1
  Divide1/1 -> [i_v]
  Relational Operator/1 -> If2/1
  [i_v] -> Relational Operator1/2, Relational Operator/2
  Relational Operator1/1 -> If2/2
  [dI_dV] -> Relational Operator1/1, Relational Operator/1

== system mppt_zero_handled/Fuzzy Logic Subsystem1/Sanitize NAN (Remove NAN and replace with 0)/If Action Subsystem ==
  In1 : Inport
  Action Port : ActionPort
  Out1 : Outport
  wires:
  In1/1 -> Out1/1

== system mppt_zero_handled/Fuzzy Logic Subsystem1/Sanitize NAN (Remove NAN and replace with 0)/If Action Subsystem1 ==
  In1 : Inport
  Action Port : ActionPort
  Out1 : Outport
  wires:
  In1/1 -> Out1/1

== system mppt_zero_handled/Incremental Condutance/When dV ==0/If Action Subsystem3 ==
  In1 : Inport
  Action Port : ActionPort
  Out1 : Outport
  wires:
  In1/1 -> Out1/1

== system mppt_zero_handled/Incremental Condutance/When dV ==0/If Action Subsystem4 ==
  In1 : Inport
  Action Port : ActionPort
  Out1 : Outport
  wires:
  In1/1 -> Out1/1

== system mppt_zero_handled/Incremental Condutance/When dV ==0/If Action Subsystem5 ==
  In1 : Inport
  Action Port : ActionPort
  Out1 : Outport
  wires:
  In1/1 -> Out1/1

== system mppt_zero_handled/Incremental Condutance/When dV ~=1/If Action Subsystem3 ==
  In1 : Inport
  Action Port : ActionPort
  Out1 : Outport
  wires:
  In1/1 -> Out1/1

== system mppt_zero_handled/Incremental Condutance/When dV ~=1/If Action Subsystem4 ==
  In1 : Inport
  Action Port : ActionPort
  Out1 : Outport
  wires:
  In1/1 -> Out1/1

== system mppt_zero_handled/Incremental Condutance/When dV ~=1/If Action Subsystem5 ==
  In1 : Inport
  Action Port : ActionPort
  Out1 : Outport
  wires:
  In1/1 -> Out1/1

== matlab function mppt_zero_handled/MATLAB Function ==
  data: v_pv input; duty_cycle output; i_pv input; delta input
function duty_cycle = mppt_i_c(v_pv, i_pv, delta)

duty_min=0;
duty_max=0.85;

persistent v_prev i_prev duty_prev;

if isempty(v_prev)
    v_prev = 0;
    i_prev = 0;
    duty_prev = 0.1;
end

dV = v_pv - v_prev;
dI = i_pv - i_prev;


%     if v_pv > 30
if dV == 0
    if dI == 0
        duty_cycle = duty_prev;
    elseif dI > 0
        duty_cycle = duty_prev + delta;
    else
        duty_cycle = duty_prev - delta;
    end
else
    if dI/dV == (-i_pv/v_pv)
        duty_cycle = duty_prev;
    elseif dI/dV > (-i_pv/v_pv)
        duty_cycle = duty_prev + delta;
    else
        duty_cycle = duty_prev - delta;
    end
end
%         duty_prev = duty_cycle;
%         v_prev = v_pv;
%         i_prev = i_pv;
%     else
%         duty_cycle = duty_prev;
%     end

%     if duty_cycle >= duty_max
%         duty_cycle = duty_max;
%     elseif duty_cycle < duty_min
%         duty_cycle = duty_min;
%     end
if duty_cycle >= duty_max || duty_cycle < duty_min
    duty_cycle = duty_prev;
end

duty_prev = duty_cycle;
v_prev = v_pv;
i_prev = i_pv;

end % end of P&O algorithm

== matlab function mppt_zero_handled/MPPT - P&O ==
  data: v_pv input; duty_cycle output; i_pv input; delta input
function duty_cycle = MPPT_PandO(v_pv,i_pv,delta)
%
duty_init=0.1;
duty_min=0;
duty_max=0.85;

persistent v_prev p_prev duty_prev;

if isempty(v_prev)
    v_prev=0;
    p_prev=0;
    duty_prev=0.1;
end

P=v_pv*i_pv;
dV=v_pv - v_prev;
dP=P - p_prev;

if dP ~=0 && v_pv>30
    if dP < 0
        if dV < 0
            duty_cycle = duty_prev - delta;
        else
            duty_cycle = duty_prev + delta;
        end
    else
        if dV < 0
            duty_cycle = duty_prev + delta;
        else
            duty_cycle = duty_prev - delta;
        end
    end
else
    duty_cycle = duty_prev;
end

if duty_cycle >= duty_max
    duty_cycle = duty_max;
elseif duty_cycle < duty_min
    duty_cycle = duty_min;
end

    
duty_prev = duty_cycle;
v_prev=v_pv;
p_prev = P;
end % end of P&O algorithm
